simulink model "Untitled1"  (R2017a)
settings: Solver=VariableStepAuto  StartTime=0.0  StopTime=10.0  RelTol=1e-3
libraries: robotlib x16
settings Model: Creator=parallels  LastModifiedBy=parallels

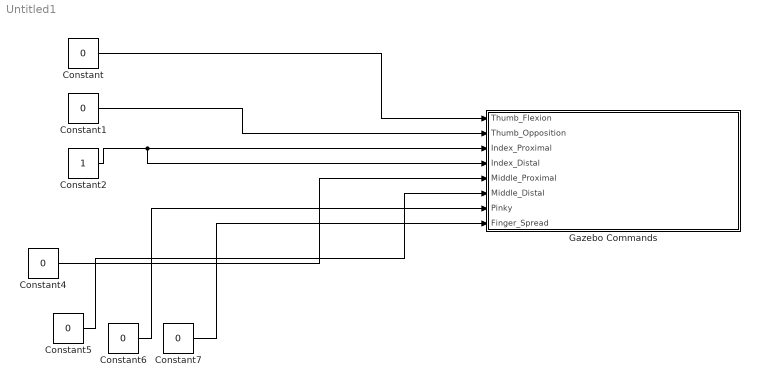
== system Untitled1 ==
  Constant{,1,4..7} (6 alike) : Constant  Value=0
  Constant2 : Constant
  Gazebo Commands : Subsystem
  wires:
  Constant/1 -> Gazebo Commands/1(Thumb_Flexion)
  Constant1/1 -> Gazebo Commands/2(Thumb_Opposition)
  Constant2/1 -> Gazebo Commands/4(Index_Distal), Gazebo Commands/3(Index_Proximal)
  Constant4/1 -> Gazebo Commands/5(Middle_Proximal)
  Constant5/1 -> Gazebo Commands/6(Middle_Distal)
  Constant6/1 -> Gazebo Commands/7(Pinky)
  Constant7/1 -> Gazebo Commands/8(Finger_Spread)

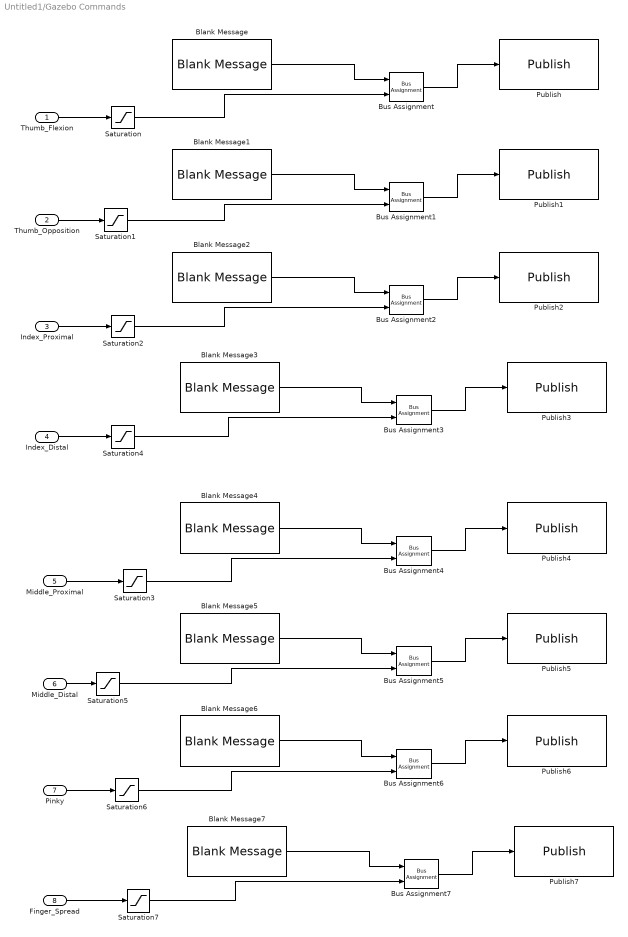
== system Untitled1/Gazebo Commands ==
  Thumb_Flexion : Inport
  Thumb_Opposition : Inport  Port=2
  Index_Proximal : Inport  Port=3
  Index_Distal : Inport  Port=4
  Middle_Proximal : Inport  Port=5
  Middle_Distal : Inport  Port=6
  Pinky : Inport  Port=7
  Finger_Spread : Inport  Port=8
  Blank Message{,1..7} (8 alike) : robotlib/Blank Message  SourceLibraryInfo=This block requires Robotics System Toolbox  messageType=std_msgs/Float64  SampleTime=inf
      settings: SourceProductBaseCode=RO
  Bus Assignment{,1..7} (8 alike) : BusAssignment  AssignedSignals=Data
  Publish : robotlib/Publish  SourceLibraryInfo=This block requires Robotics System Toolbox  topicSource=Select from ROS network  topic=/svh_controller/Thumb_Flexion  messageType=std_msgs/Float64  messageQueueLength=1
      settings: SourceProductBaseCode=RO
  Publish1 : robotlib/Publish  SourceLibraryInfo=This block requires Robotics System Toolbox  topicSource=Select from ROS network  topic=/svh_controller/Thumb_Opposition  messageType=std_msgs/Float64  messageQueueLength=1
      settings: SourceProductBaseCode=RO
  Publish2 : robotlib/Publish  SourceLibraryInfo=This block requires Robotics System Toolbox  topicSource=Select from ROS network  topic=/svh_controller/Index_Proximal  messageType=std_msgs/Float64  messageQueueLength=1
      settings: SourceProductBaseCode=RO
  Publish3 : robotlib/Publish  SourceLibraryInfo=This block requires Robotics System Toolbox  topicSource=Select from ROS network  topic=/svh_controller/Index_Distal  messageType=std_msgs/Float64  messageQueueLength=1
      settings: SourceProductBaseCode=RO
  Publish4 : robotlib/Publish  SourceLibraryInfo=This block requires Robotics System Toolbox  topicSource=Specify your own  topic=/svh_controller/Middle_Proximal  messageType=std_msgs/Float64  messageQueueLength=1
      settings: SourceProductBaseCode=RO
  Publish5 : robotlib/Publish  SourceLibraryInfo=This block requires Robotics System Toolbox  topicSource=Specify your own  topic=/svh_controller/Middle_Distal  messageType=std_msgs/Float64  messageQueueLength=1
      settings: SourceProductBaseCode=RO
  Publish6 : robotlib/Publish  SourceLibraryInfo=This block requires Robotics System Toolbox  topicSource=Specify your own  topic=/svh_controller/Pinky  messageType=std_msgs/Float64  messageQueueLength=1
      settings: SourceProductBaseCode=RO
  Publish7 : robotlib/Publish  SourceLibraryInfo=This block requires Robotics System Toolbox  topicSource=Specify your own  topic=/svh_controller/Finger_Spread  messageType=std_msgs/Float64  messageQueueLength=1
      settings: SourceProductBaseCode=RO
  Saturation : Saturate  UpperLimit=0.9704  LowerLimit=0
  Saturation1 : Saturate  UpperLimit=0.9879  LowerLimit=-0.0
  Saturation2 : Saturate  UpperLimit=0.79849  LowerLimit=0
  Saturation3 : Saturate  UpperLimit=0.79849  LowerLimit=0
  Saturation4 : Saturate  UpperLimit=1.334  LowerLimit=0
  Saturation5 : Saturate  UpperLimit=1.334  LowerLimit=0
  Saturation6 : Saturate  UpperLimit=0.9704  LowerLimit=0
  Saturation7 : Saturate  UpperLimit=0.5829  LowerLimit=0
  wires:
  Bus Assignment/1 -> Publish/1
  Blank Message/1 -> Bus Assignment/1
  Blank Message2/1 -> Bus Assignment2/1
  Blank Message3/1 -> Bus Assignment3/1
  Index_Proximal/1 -> Saturation2/1
  Thumb_Flexion/1 -> Saturation/1
  Blank Message1/1 -> Bus Assignment1/1
  Index_Distal/1 -> Saturation4/1
  Bus Assignment2/1 -> Publish2/1
  Thumb_Opposition/1 -> Saturation1/1
  Bus Assignment3/1 -> Publish3/1
  Bus Assignment1/1 -> Publish1/1
  Bus Assignment4/1 -> Publish4/1
  Blank Message5/1 -> Bus Assignment5/1
  Middle_Distal/1 -> Saturation5/1
  Bus Assignment5/1 -> Publish5/1
  Blank Message7/1 -> Bus Assignment7/1
  Bus Assignment7/1 -> Publish7/1
  Bus Assignment6/1 -> Publish6/1
  Finger_Spread/1 -> Saturation7/1
  Middle_Proximal/1 -> Saturation3/1
  Pinky/1 -> Saturation6/1
  Blank Message6/1 -> Bus Assignment6/1
  Blank Message4/1 -> Bus Assignment4/1
  Saturation1/1 -> Bus Assignment1/2
  Saturation/1 -> Bus Assignment/2
  Saturation2/1 -> Bus Assignment2/2
  Saturation3/1 -> Bus Assignment4/2
  Saturation4/1 -> Bus Assignment3/2
  Saturation5/1 -> Bus Assignment5/2
  Saturation6/1 -> Bus Assignment6/2
  Saturation7/1 -> Bus Assignment7/2
